simulink model "Real_RPU"  (R2016b)
settings: Solver=FixedStepAuto  StartTime=0.0  StopTime=inf  FixedStep=RealRPU.tiSimnTiStep_C  RelTol=1e-3  SampleTimeConstraint=STIndependent  EnableMultiTasking=on
settings Model: Creator=m01wolf  LastModifiedBy=bunver
settings DataIOCC: SaveFormat=StructureWithTime  SaveOutput=off  DSMLogging=off  VisualizeSimOutput=off  SaveTime=off  SignalLoggingName=Results
settings OptimizationCC: BlockReduction=off  ConditionallyExecuteInputs=off  LifeSpan=inf
settings DebuggingCC: AllowSymbolicDim=off  SFUnexpectedBacktrackingDiag=warning  SFNoUnconditionalDefaultTransitionDiag=warning  SFExecutionAtInitializationDiag=none
settings ModelReferenceCC: ModelReferenceNumInstancesAllowed=Single  PropagateSignalLabelsOutOfModel=off
settings GRTTargetCC: TargetLangStandard=C89/C90 (ANSI)
settings ConfigComp: CovMetricSettings=dw  CovHtmlReporting=on  CovSaveCumulativeToWorkspaceVar=on  CovSaveSingleToWorkspaceVar=on  CovExternalEMLEnable=off

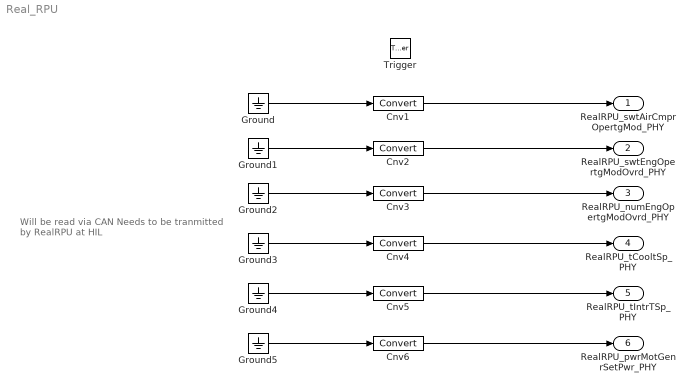
== system Real_RPU ==
  note: Will be read via CAN
      | Needs to be tranmitted by RealRPU at HIL
  Trigger : TriggerPort  TriggerType=function-call  VariantControl=Variant  PortDimensions=1
  Cnv{1..6} (6 alike) : DataTypeConversion
  Ground{,1..5} (6 alike) : Ground
  RealRPU_swtAirCmprOpertgMod_PHY : Outport
  RealRPU_swtEngOpertgModOvrd_PHY : Outport  Port=2
  RealRPU_numEngOpertgModOvrd_PHY : Outport  Port=3
  RealRPU_tCooltSp_PHY : Outport  Port=4
  RealRPU_tIntrTSp_PHY : Outport  Port=5
  RealRPU_pwrMotGenrSetPwr_PHY : Outport  Port=6
  wires:
  Cnv1/1 -> RealRPU_swtAirCmprOpertgMod_PHY/1
  Cnv2/1 -> RealRPU_swtEngOpertgModOvrd_PHY/1
  Cnv3/1 -> RealRPU_numEngOpertgModOvrd_PHY/1
  Cnv4/1 -> RealRPU_tCooltSp_PHY/1
  Cnv5/1 -> RealRPU_tIntrTSp_PHY/1
  Cnv6/1 -> RealRPU_pwrMotGenrSetPwr_PHY/1
  Ground/1 -> Cnv1/1
  Ground1/1 -> Cnv2/1
  Ground2/1 -> Cnv3/1
  Ground3/1 -> Cnv4/1
  Ground4/1 -> Cnv5/1
  Ground5/1 -> Cnv6/1
